simulink model "braccio_test"  (R2021a)
settings: Solver=FixedStepAuto  StartTime=0.0  StopTime=inf  RelTol=1e-3  EnableMultiTasking=on
libraries: arduinolib x7
settings Model: SILPILModeSetting=veronly  ExtModeTrigDuration=2  Creator=angelo  LastModifiedBy=angelo
settings OptimizationCC: EnhancedBackFolding=on  PassReuseOutputArgsAs=Individual arguments  ZeroExternalMemoryAtStartup=off  ZeroInternalMemoryAtStartup=off  MaxStackSize=64  OptimizeBlockOrder=speed  DifferentSizesBufferReuse=on  OptimizationCustomize=off  EfficientTunableParamExpr=on
settings DebuggingCC: ParameterTunabilityLossMsg=error
settings HardwareCC: ProdBitPerInt=16  ProdBitPerPointer=16  ProdBitPerSizeT=16  ProdBitPerPtrDiffT=16  ProdLargestAtomicFloat=None  ProdWordSize=8  ProdHWDeviceType=Atmel->AVR
settings SFSimCC: MATLABDynamicMemAlloc=off
settings RTWCC: SystemTargetFile=ert.tlc  HardwareBoard=Arduino Uno  TemplateMakefile=ert_default_tmf  Toolchain=Arduino AVR  BuildConfiguration=Faster Runs
settings CodeAppCC: ForceParamTrailComments=on  IgnoreCustomStorageClasses=off  OperatorAnnotations=on  SimulinkDataObjDesc=on  SFDataObjDesc=on  InsertBlockDesc=on
settings ERTTargetCC: SupportContinuousTime=on  SupportVariableSizeSignals=on  ExtModeStaticAllocSize=250

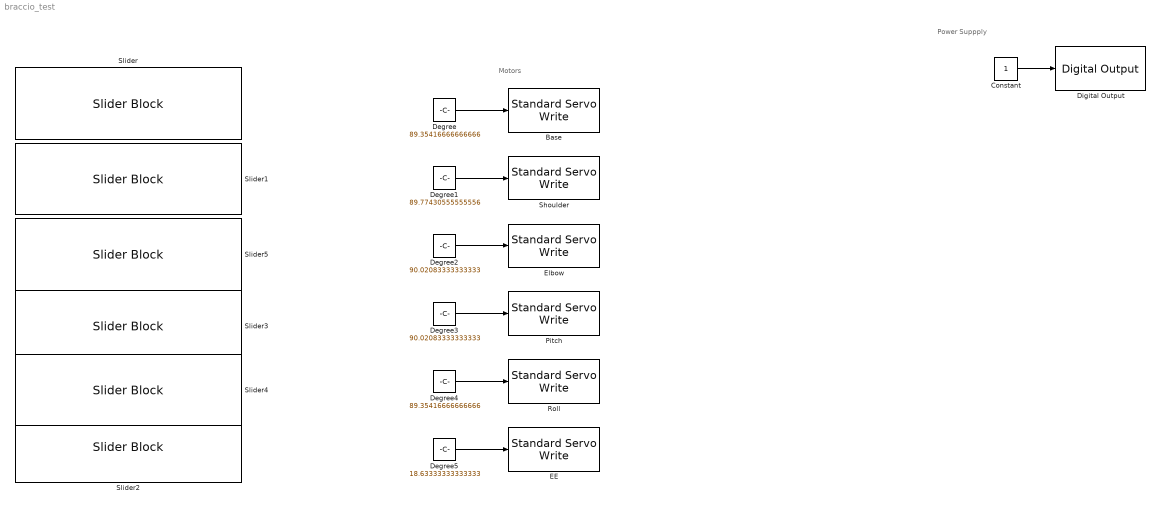
== system braccio_test ==
  note: Motors
  note: Power Suppply
  Base : arduinolib/Standard Servo Write  pinNumber=11  ServoIndex=0  blockPlatform=ARDUINO
  Constant : Constant
  Degree : Constant  Value=89.35416666666666
  Degree1 : Constant  Value=89.77430555555556
  Degree2 : Constant  Value=90.02083333333333
  Degree3 : Constant  Value=90.02083333333333
  Degree4 : Constant  Value=89.35416666666666
  Degree5 : Constant  Value=18.63333333333333
  Digital Output : arduinolib/Digital Output  pinNumber=12  Direction=output  blockPlatform=arduino
  EE : arduinolib/Standard Servo Write  pinNumber=3  ServoIndex=1  blockPlatform=ARDUINO
  Elbow : arduinolib/Standard Servo Write  pinNumber=9  ServoIndex=2  blockPlatform=ARDUINO
  Pitch : arduinolib/Standard Servo Write  pinNumber=6  ServoIndex=3  blockPlatform=ARDUINO
  Roll : arduinolib/Standard Servo Write  pinNumber=5  ServoIndex=4  blockPlatform=ARDUINO
  Shoulder : arduinolib/Standard Servo Write  pinNumber=10  ServoIndex=5  blockPlatform=ARDUINO
  Slider{,3..5} (4 alike) : SliderBlock  ScaleMax=180
  Slider1 : SliderBlock  ScaleMin=15  ScaleMax=165
  Slider2 : SliderBlock  ScaleMin=10  ScaleMax=73
  wires:
  Constant/1 -> Digital Output/1
  Degree/1 -> Base/1
  Degree5/1 -> EE/1
  Degree2/1 -> Elbow/1
  Degree3/1 -> Pitch/1
  Degree4/1 -> Roll/1
  Degree1/1 -> Shoulder/1
